simulink model "PI_Controller_with_SupFuzzy_TF"  (R2018b)
settings: Solver=VariableStepAuto  StartTime=0.0  StopTime=50  RelTol=1e-3
settings Model: Creator=admin  LastModifiedBy=admin

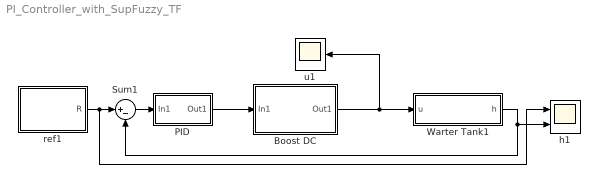
== system PI_Controller_with_SupFuzzy_TF ==
  Boost DC : Subsystem
  PID : Subsystem  mask{Kp1=0.11, Kd1=0, Ki1=1.1}
  Sum1 : Sum  Inputs=|+-
  Warter Tank1 : Subsystem  mask{h0=10, Ah=100, k=300, Cd=0.6, a=1, g=981}
      mask prompts: h0 "Do cao ban dau (cm)"; Ah "Tiet dien ngang bon chua (cm2)"; k "He so ty le cong suat may bom"; Cd "He so xa"; a "Tiet dien van xa"; g "Gia toc trong truong"
  h1 : Scope  NumInputPorts=2
  ref1 : Subsystem
  u1 : Scope
  wires:
  Warter Tank1/1(h) -> Sum1/2, h1/2
  ref1/1(R) -> h1/1, Sum1/1
  Sum1/1 -> PID/1(In1)
  Boost DC/1(Out1) -> Warter Tank1/1(u), u1/1
  PID/1(Out1) -> Boost DC/1(In1)

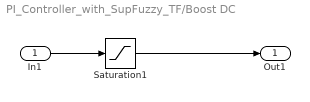
== system PI_Controller_with_SupFuzzy_TF/Boost DC ==
  In1 : Inport
  Saturation1 : Saturate  UpperLimit=36  LowerLimit=0
  Out1 : Outport
  wires:
  Saturation1/1 -> Out1/1
  In1/1 -> Saturation1/1

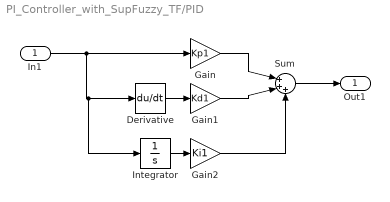
== system PI_Controller_with_SupFuzzy_TF/PID ==
  In1 : Inport
  Derivative : Derivative
  Gain : Gain  Gain=Kp1
  Gain1 : Gain  Gain=Kd1
  Gain2 : Gain  Gain=Ki1
  Integrator : Integrator
  Sum : Sum  Inputs=|+++
  Out1 : Outport
  wires:
  Sum/1 -> Out1/1
  Gain2/1 -> Sum/3
  Gain/1 -> Sum/1
  Gain1/1 -> Sum/2
  Integrator/1 -> Gain2/1
  Derivative/1 -> Gain1/1
  In1/1 -> Gain/1, Derivative/1, Integrator/1

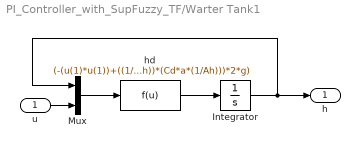
== system PI_Controller_with_SupFuzzy_TF/Warter Tank1 ==
  u : Inport
  Integrator : Integrator  InitialCondition=h0  LimitOutput=on  UpperSaturationLimit=100  LowerSaturationLimit=0
  Mux : Mux  Inputs=2
  hd : Fcn  Expr=(-(u(1)*u(1))+((1/Ah)*k)*((1/Ah)*k)*u(2)*u(2))/(((Cd*a*(1/Ah))*(Cd*a*(1/Ah)))*2*g)
  h : Outport
  wires:
  hd/1 -> Integrator/1
  Integrator/1 -> Mux/1, h/1
  u/1 -> Mux/2
  Mux/1 -> hd/1

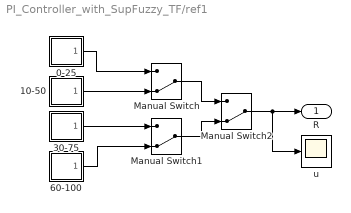
== system PI_Controller_with_SupFuzzy_TF/ref1 ==
  0-25 : Subsystem
  10-50 : Subsystem
  30-75 : Subsystem
  60-100 : Subsystem
  Manual Switch : ManualSwitch  CurrentSetting=0
  Manual Switch1 : ManualSwitch  CurrentSetting=0
  Manual Switch2 : ManualSwitch  CurrentSetting=0
  u : Scope
  R : Outport
  wires:
  Manual Switch/1 -> Manual Switch2/1
  Manual Switch1/1 -> Manual Switch2/2
  Manual Switch2/1 -> u/1, R/1
  10-50/1(Out1) -> Manual Switch/2
  0-25/1(Out1) -> Manual Switch/1
  30-75/1(Out1) -> Manual Switch1/1
  60-100/1(Out1) -> Manual Switch1/2

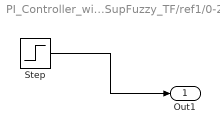
== system PI_Controller_with_SupFuzzy_TF/ref1/0-25 ==
  Step : Step  Time=3  After=25  SampleTime=0
  Out1 : Outport
  wires:
  Step/1 -> Out1/1

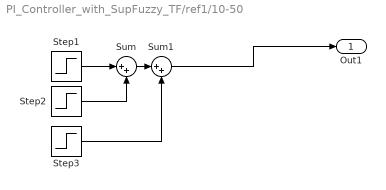
== system PI_Controller_with_SupFuzzy_TF/ref1/10-50 ==
  Step1 : Step  Time=3  After=10  SampleTime=0
  Step2 : Step  Time=6  After=20  SampleTime=0
  Step3 : Step  Time=9  After=20  SampleTime=0
  Sum : Sum  Inputs=|++
  Sum1 : Sum  Inputs=|++
  Out1 : Outport
  wires:
  Sum/1 -> Sum1/1
  Step1/1 -> Sum/1
  Sum1/1 -> Out1/1
  Step3/1 -> Sum1/2
  Step2/1 -> Sum/2

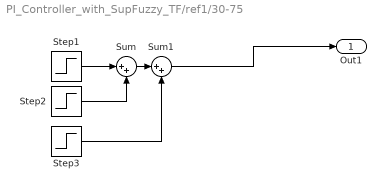
== system PI_Controller_with_SupFuzzy_TF/ref1/30-75 ==
  Step1 : Step  Time=3  After=30  SampleTime=0
  Step2 : Step  Time=6  After=30  SampleTime=0
  Step3 : Step  Time=9  After=15  SampleTime=0
  Sum : Sum  Inputs=|++
  Sum1 : Sum  Inputs=|++
  Out1 : Outport
  wires:
  Sum/1 -> Sum1/1
  Step1/1 -> Sum/1
  Sum1/1 -> Out1/1
  Step3/1 -> Sum1/2
  Step2/1 -> Sum/2

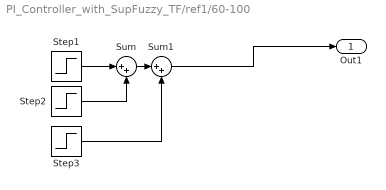
== system PI_Controller_with_SupFuzzy_TF/ref1/60-100 ==
  Step1 : Step  Time=3  After=60  SampleTime=0
  Step2 : Step  Time=6  After=20  SampleTime=0
  Step3 : Step  Time=9  After=20  SampleTime=0
  Sum : Sum  Inputs=|++
  Sum1 : Sum  Inputs=|++
  Out1 : Outport
  wires:
  Sum/1 -> Sum1/1
  Step1/1 -> Sum/1
  Sum1/1 -> Out1/1
  Step3/1 -> Sum1/2
  Step2/1 -> Sum/2
